simulink model "twoNodeTether_th"  (R2018b)
settings: Solver=VariableStepAuto  StartTime=0.0  StopTime=0  RelTol=1e-3
values from neighbouring files (symbols this model uses):
  airNodePos = [0 0 1]'    [twoNodeTether_ts.m]
  airNodeVel = [0 0 0]'    [twoNodeTether_ts.m]
  flowVec = [1 0 0]'    [twoNodeTether_ts.m]
  gndNodePos = [0 0 0]'    [twoNodeTether_ts.m]
  gndNodeVel = [0 0 0]'    [twoNodeTether_ts.m]
  unstretchedLength = 1    [nodeNetBuoyFrc.m]    (also in twoNodeTether_ts.m = norm(airNodePos(:)-gndNodePos(:)))
libraries: twoNodeTether_cl x1
settings Model: Creator=mcobb  LastModifiedBy=mcobb

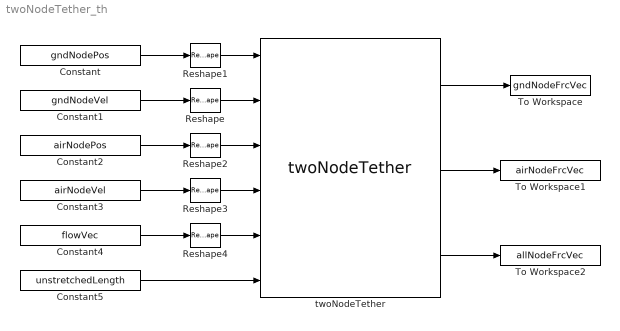
== system twoNodeTether_th ==
  Constant : Constant  Value=gndNodePos
  Constant1 : Constant  Value=gndNodeVel
  Constant2 : Constant  Value=airNodePos
  Constant3 : Constant  Value=airNodeVel
  Constant4 : Constant  Value=flowVec
  Constant5 : Constant  Value=unstretchedLength
  Reshape{,1..4} (5 alike) : Reshape  OutputDimensionality=Column vector (2-D)
  To Workspace : ToWorkspace  VariableName=gndNodeFrcVec  SaveFormat=Timeseries  SampleTime=-1
  To Workspace1 : ToWorkspace  VariableName=airNodeFrcVec  SaveFormat=Timeseries  SampleTime=-1
  To Workspace2 : ToWorkspace  VariableName=allNodeFrcVec  SaveFormat=Timeseries  SampleTime=-1
  twoNodeTether : twoNodeTether_cl/twoNodeTether  thr=thr  flowDensity=1  gravity=9.81  numNodes=2
  wires:
  Constant/1 -> Reshape1/1
  Constant1/1 -> Reshape/1
  Constant2/1 -> Reshape2/1
  Constant3/1 -> Reshape3/1
  Constant4/1 -> Reshape4/1
  Constant5/1 -> twoNodeTether/6
  twoNodeTether/1 -> To Workspace/1
  twoNodeTether/2 -> To Workspace1/1
  Reshape1/1 -> twoNodeTether/1
  Reshape/1 -> twoNodeTether/2
  Reshape2/1 -> twoNodeTether/3
  Reshape3/1 -> twoNodeTether/4
  Reshape4/1 -> twoNodeTether/5
  twoNodeTether/3 -> To Workspace2/1
